simulink model "uuv_depth_control"  (R2021a)
settings: Solver=ode1  StartTime=0  StopTime=1000  FixedStep=0.1  RelTol=1e-3
undefined symbols (not defined in the file or in its folder): sigbuilder_block
(part 2 of 2)

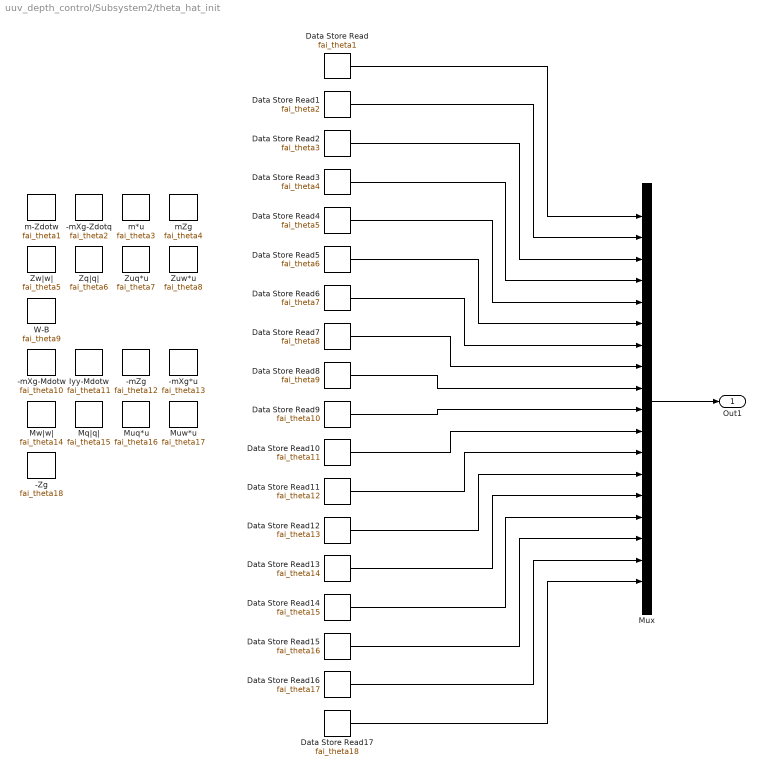
== system uuv_depth_control/Subsystem2/theta_hat_init ==
  -Zg : DataStoreMemory  DataStoreName=fai_theta18  ReadBeforeWriteMsg=warning  WriteAfterWriteMsg=warning  WriteAfterReadMsg=warning  InitialValue=-0.0196000000000000  ShowAdditionalParam=off
  -mXg*u : DataStoreMemory  DataStoreName=fai_theta13  ReadBeforeWriteMsg=warning  WriteAfterWriteMsg=warning  WriteAfterReadMsg=warning  ShowAdditionalParam=off
  -mXg-Mdotw : DataStoreMemory  DataStoreName=fai_theta10  ReadBeforeWriteMsg=warning  WriteAfterWriteMsg=warning  WriteAfterReadMsg=warning  InitialValue=1.93000000000000  ShowAdditionalParam=off
  -mXg-Zdotq : DataStoreMemory  DataStoreName=fai_theta2  ReadBeforeWriteMsg=warning  WriteAfterWriteMsg=warning  WriteAfterReadMsg=warning  InitialValue=1.930000000000000  ShowAdditionalParam=off
  -mZg : DataStoreMemory  DataStoreName=fai_theta12  ReadBeforeWriteMsg=warning  WriteAfterWriteMsg=warning  WriteAfterReadMsg=warning  InitialValue=-0.597408000000000  ShowAdditionalParam=off
  Data Store Read : DataStoreRead  DataStoreName=fai_theta1  IndexOptions=Index vector (dialog)  Indices=1  OutputSizes=1
  Data Store Read1 : DataStoreRead  DataStoreName=fai_theta2  IndexOptions=Index vector (dialog)  Indices=1  OutputSizes=1
  Data Store Read10 : DataStoreRead  DataStoreName=fai_theta11  IndexOptions=Index vector (dialog)  Indices=1  OutputSizes=1
  Data Store Read11 : DataStoreRead  DataStoreName=fai_theta12  IndexOptions=Index vector (dialog)  Indices=1  OutputSizes=1
  Data Store Read12 : DataStoreRead  DataStoreName=fai_theta13  IndexOptions=Index vector (dialog)  Indices=1  OutputSizes=1
  Data Store Read13 : DataStoreRead  DataStoreName=fai_theta14  IndexOptions=Index vector (dialog)  Indices=1  OutputSizes=1
  Data Store Read14 : DataStoreRead  DataStoreName=fai_theta15  IndexOptions=Index vector (dialog)  Indices=1  OutputSizes=1
  Data Store Read15 : DataStoreRead  DataStoreName=fai_theta16  IndexOptions=Index vector (dialog)  Indices=1  OutputSizes=1
  Data Store Read16 : DataStoreRead  DataStoreName=fai_theta17  IndexOptions=Index vector (dialog)  Indices=1  OutputSizes=1
  Data Store Read17 : DataStoreRead  DataStoreName=fai_theta18  IndexOptions=Index vector (dialog)  Indices=1  OutputSizes=1
  Data Store Read2 : DataStoreRead  DataStoreName=fai_theta3  IndexOptions=Index vector (dialog)  Indices=1  OutputSizes=1
  Data Store Read3 : DataStoreRead  DataStoreName=fai_theta4  IndexOptions=Index vector (dialog)  Indices=1  OutputSizes=1
  Data Store Read4 : DataStoreRead  DataStoreName=fai_theta5  IndexOptions=Index vector (dialog)  Indices=1  OutputSizes=1
  Data Store Read5 : DataStoreRead  DataStoreName=fai_theta6  IndexOptions=Index vector (dialog)  Indices=1  OutputSizes=1
  Data Store Read6 : DataStoreRead  DataStoreName=fai_theta7  IndexOptions=Index vector (dialog)  Indices=1  OutputSizes=1
  Data Store Read7 : DataStoreRead  DataStoreName=fai_theta8  IndexOptions=Index vector (dialog)  Indices=1  OutputSizes=1
  Data Store Read8 : DataStoreRead  DataStoreName=fai_theta9  IndexOptions=Index vector (dialog)  Indices=1  OutputSizes=1
  Data Store Read9 : DataStoreRead  DataStoreName=fai_theta10  IndexOptions=Index vector (dialog)  Indices=1  OutputSizes=1
  Iyy-Mdotw : DataStoreMemory  DataStoreName=fai_theta11  ReadBeforeWriteMsg=warning  WriteAfterWriteMsg=warning  WriteAfterReadMsg=warning  InitialValue=8.330000000000000  ShowAdditionalParam=off
  Mq|q| : DataStoreMemory  DataStoreName=fai_theta15  ReadBeforeWriteMsg=warning  WriteAfterWriteMsg=warning  WriteAfterReadMsg=warning  InitialValue=-9.40000000000000  ShowAdditionalParam=off
  Muq*u : DataStoreMemory  DataStoreName=fai_theta16  ReadBeforeWriteMsg=warning  WriteAfterWriteMsg=warning  WriteAfterReadMsg=warning  InitialValue=-1  ShowAdditionalParam=off
  Muw*u : DataStoreMemory  DataStoreName=fai_theta17  ReadBeforeWriteMsg=warning  WriteAfterWriteMsg=warning  WriteAfterReadMsg=warning  InitialValue=12  ShowAdditionalParam=off
  Mux : Mux  Inputs=18
  Mw|w| : DataStoreMemory  DataStoreName=fai_theta14  ReadBeforeWriteMsg=warning  WriteAfterWriteMsg=warning  WriteAfterReadMsg=warning  InitialValue=3.18000000000000  ShowAdditionalParam=off
  W-B : DataStoreMemory  DataStoreName=fai_theta9  ReadBeforeWriteMsg=warning  WriteAfterWriteMsg=warning  WriteAfterReadMsg=warning  InitialValue=-9  ShowAdditionalParam=off
  Zq|q| : DataStoreMemory  DataStoreName=fai_theta6  ReadBeforeWriteMsg=warning  WriteAfterWriteMsg=warning  WriteAfterReadMsg=warning  InitialValue=-0.632000000000000  ShowAdditionalParam=off
  Zuq*u : DataStoreMemory  DataStoreName=fai_theta7  ReadBeforeWriteMsg=warning  WriteAfterWriteMsg=warning  WriteAfterReadMsg=warning  InitialValue=-2.61000000000000  ShowAdditionalParam=off
  Zuw*u : DataStoreMemory  DataStoreName=fai_theta8  ReadBeforeWriteMsg=warning  WriteAfterWriteMsg=warning  WriteAfterReadMsg=warning  InitialValue=-14.3000000000000  ShowAdditionalParam=off
  Zw|w| : DataStoreMemory  DataStoreName=fai_theta5  ReadBeforeWriteMsg=warning  WriteAfterWriteMsg=warning  WriteAfterReadMsg=warning  InitialValue=-131  ShowAdditionalParam=off
  m*u : DataStoreMemory  DataStoreName=fai_theta3  ReadBeforeWriteMsg=warning  WriteAfterWriteMsg=warning  WriteAfterReadMsg=warning  InitialValue=15.2400000000000  ShowAdditionalParam=off
  m-Zdotw : DataStoreMemory  DataStoreName=fai_theta1  ReadBeforeWriteMsg=warning  WriteAfterWriteMsg=warning  WriteAfterReadMsg=warning  InitialValue=65.980000000000000  ShowAdditionalParam=off
  mZg : DataStoreMemory  DataStoreName=fai_theta4  ReadBeforeWriteMsg=warning  WriteAfterWriteMsg=warning  WriteAfterReadMsg=warning  InitialValue=0.597408000000000  ShowAdditionalParam=off
  Out1 : Outport
  wires:
  Mux/1 -> Out1/1
  Data Store Read/1 -> Mux/1
  Data Store Read3/1 -> Mux/4
  Data Store Read8/1 -> Mux/9
  Data Store Read5/1 -> Mux/6
  Data Store Read10/1 -> Mux/11
  Data Store Read4/1 -> Mux/5
  Data Store Read15/1 -> Mux/16
  Data Store Read12/1 -> Mux/13
  Data Store Read1/1 -> Mux/2
  Data Store Read14/1 -> Mux/15
  Data Store Read9/1 -> Mux/10
  Data Store Read7/1 -> Mux/8
  Data Store Read13/1 -> Mux/14
  Data Store Read2/1 -> Mux/3
  Data Store Read6/1 -> Mux/7
  Data Store Read17/1 -> Mux/18
  Data Store Read11/1 -> Mux/12
  Data Store Read16/1 -> Mux/17

== system uuv_depth_control/Subsystem4/cmd ==
  Add : Sum
  Cmd Depth : Subsystem  Tag=STV Subsys  LoadFcn=sigbuilder_block('load');  StartFcn=sigbuilder_block('start');  StopFcn=sigbuilder_block('stop');  ClipboardFcn=sigbuilder_block('clipboard');  mask(Sigbuilder block){tuvar=[0:10]}
      mask help: Simulink:masks:SigbuilderBlock_MD
      mask init:
      | if ~strcmp(get_param(bdroot(gcbh),'SimulationStatus'),'stopped') tuvar = sigbuilder_block('maskInit'); end
      settings: CopyFcn=sigbuilder_block('copy');  DeleteFcn=sigbuilder_block('delete');  ModelCloseFcn=sigbuilder_block('modelClose');  PreSaveFcn=sigbuilder_block('preSave');  PauseFcn=sigbuilder_block('pause');  ContinueFcn=sigbuilder_block('continue');  NameChangeFcn=sigbuilder_block('namechange');  OpenFcn=sigbuilder_block('open',[361.8 75 550.8 375 ]);  CloseFcn=sigbuilder_block('close');
      mask Display: plot(0, 0, 100, 100,[2, 2, 32, 32, 2], [68, 8, 8, 68, 68],[32, 2], [38, 38], [32, 19, 2],[53, 60, 44], [32, 17, 17, 2],[16, 16, 31, 31]);txt = getActiveGroup(gcbh);text(2, 100, txt,'verticalAlignment', 'top');
  Cmd theta : Subsystem  Tag=STV Subsys  LoadFcn=sigbuilder_block('load');  StartFcn=sigbuilder_block('start');  StopFcn=sigbuilder_block('stop');  ClipboardFcn=sigbuilder_block('clipboard');  mask(Sigbuilder block){tuvar=[0:10]}
      mask help: Simulink:masks:SigbuilderBlock_MD
      mask init:
      | if ~strcmp(get_param(bdroot(gcbh),'SimulationStatus'),'stopped') tuvar = sigbuilder_block('maskInit'); end
      settings: CopyFcn=sigbuilder_block('copy');  DeleteFcn=sigbuilder_block('delete');  ModelCloseFcn=sigbuilder_block('modelClose');  PreSaveFcn=sigbuilder_block('preSave');  PauseFcn=sigbuilder_block('pause');  ContinueFcn=sigbuilder_block('continue');  NameChangeFcn=sigbuilder_block('namechange');  OpenFcn=sigbuilder_block('open',[313.2 49.2 550.8 400.8 ]);  CloseFcn=sigbuilder_block('close');
      mask Display: plot(0, 0, 100, 100,[2, 2, 32, 32, 2], [68, 8, 8, 68, 68],[32, 2], [38, 38], [32, 19, 2],[53, 60, 44], [32, 17, 17, 2],[16, 16, 31, 31]);txt = getActiveGroup(gcbh);text(2, 100, txt,'verticalAlignment', 'top');
  Constant1 : Constant  Value=-1
  Constant2 : Constant  Value=0
  Constant3 : Constant
  Constant4 : Constant  Value=0
  Signal Generator : SignalGenerator  Amplitude=3  Frequency=0.1  Units=rad/sec
  Switch : Switch  Criteria=u2 > Threshold
  Switch1 : Switch  Criteria=u2 > Threshold
  Out1 : Outport
  Out2 : Outport  Port=2
  wires:
  Cmd Depth/1(Signal 2) -> Add/2
  Cmd theta/1(Signal 1) -> Switch1/1
  Signal Generator/1 -> Switch/1
  Add/1 -> Out1/1  "cmd_z"
  Constant4/1 -> Switch/3
  Switch/1 -> Add/1
  Constant1/1 -> Switch/2
  Constant2/1 -> Switch1/3
  Constant3/1 -> Switch1/2
  Switch1/1 -> Out2/1  "cmd_theta"

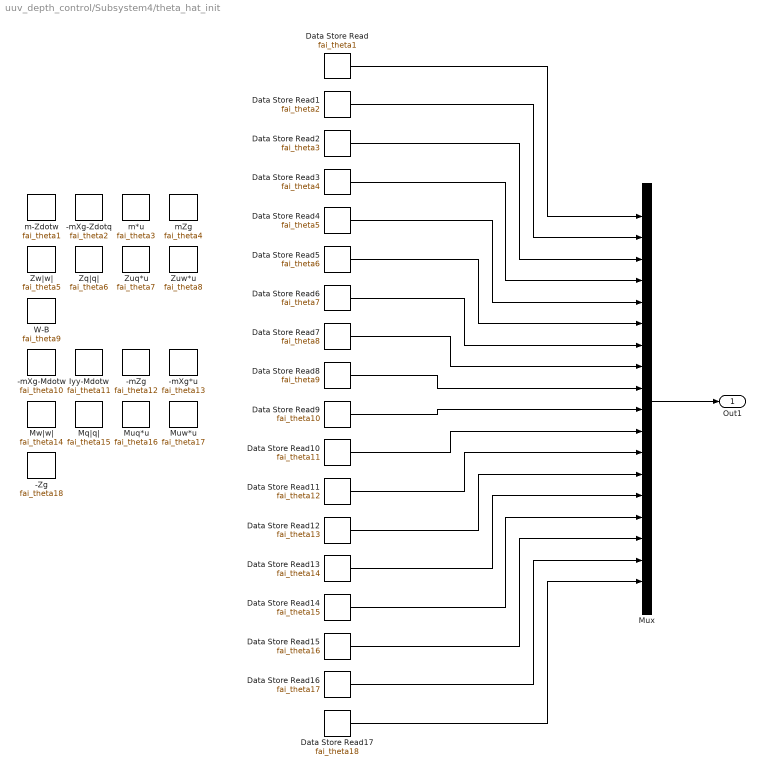
== system uuv_depth_control/Subsystem4/theta_hat_init ==
  -Zg : DataStoreMemory  DataStoreName=fai_theta18  ReadBeforeWriteMsg=warning  WriteAfterWriteMsg=warning  WriteAfterReadMsg=warning  InitialValue=-0.0196000000000000  ShowAdditionalParam=off
  -mXg*u : DataStoreMemory  DataStoreName=fai_theta13  ReadBeforeWriteMsg=warning  WriteAfterWriteMsg=warning  WriteAfterReadMsg=warning  ShowAdditionalParam=off
  -mXg-Mdotw : DataStoreMemory  DataStoreName=fai_theta10  ReadBeforeWriteMsg=warning  WriteAfterWriteMsg=warning  WriteAfterReadMsg=warning  InitialValue=1.93000000000000  ShowAdditionalParam=off
  -mXg-Zdotq : DataStoreMemory  DataStoreName=fai_theta2  ReadBeforeWriteMsg=warning  WriteAfterWriteMsg=warning  WriteAfterReadMsg=warning  InitialValue=1.930000000000000  ShowAdditionalParam=off
  -mZg : DataStoreMemory  DataStoreName=fai_theta12  ReadBeforeWriteMsg=warning  WriteAfterWriteMsg=warning  WriteAfterReadMsg=warning  InitialValue=-0.597408000000000  ShowAdditionalParam=off
  Data Store Read : DataStoreRead  DataStoreName=fai_theta1  IndexOptions=Index vector (dialog)  Indices=1  OutputSizes=1
  Data Store Read1 : DataStoreRead  DataStoreName=fai_theta2  IndexOptions=Index vector (dialog)  Indices=1  OutputSizes=1
  Data Store Read10 : DataStoreRead  DataStoreName=fai_theta11  IndexOptions=Index vector (dialog)  Indices=1  OutputSizes=1
  Data Store Read11 : DataStoreRead  DataStoreName=fai_theta12  IndexOptions=Index vector (dialog)  Indices=1  OutputSizes=1
  Data Store Read12 : DataStoreRead  DataStoreName=fai_theta13  IndexOptions=Index vector (dialog)  Indices=1  OutputSizes=1
  Data Store Read13 : DataStoreRead  DataStoreName=fai_theta14  IndexOptions=Index vector (dialog)  Indices=1  OutputSizes=1
  Data Store Read14 : DataStoreRead  DataStoreName=fai_theta15  IndexOptions=Index vector (dialog)  Indices=1  OutputSizes=1
  Data Store Read15 : DataStoreRead  DataStoreName=fai_theta16  IndexOptions=Index vector (dialog)  Indices=1  OutputSizes=1
  Data Store Read16 : DataStoreRead  DataStoreName=fai_theta17  IndexOptions=Index vector (dialog)  Indices=1  OutputSizes=1
  Data Store Read17 : DataStoreRead  DataStoreName=fai_theta18  IndexOptions=Index vector (dialog)  Indices=1  OutputSizes=1
  Data Store Read2 : DataStoreRead  DataStoreName=fai_theta3  IndexOptions=Index vector (dialog)  Indices=1  OutputSizes=1
  Data Store Read3 : DataStoreRead  DataStoreName=fai_theta4  IndexOptions=Index vector (dialog)  Indices=1  OutputSizes=1
  Data Store Read4 : DataStoreRead  DataStoreName=fai_theta5  IndexOptions=Index vector (dialog)  Indices=1  OutputSizes=1
  Data Store Read5 : DataStoreRead  DataStoreName=fai_theta6  IndexOptions=Index vector (dialog)  Indices=1  OutputSizes=1
  Data Store Read6 : DataStoreRead  DataStoreName=fai_theta7  IndexOptions=Index vector (dialog)  Indices=1  OutputSizes=1
  Data Store Read7 : DataStoreRead  DataStoreName=fai_theta8  IndexOptions=Index vector (dialog)  Indices=1  OutputSizes=1
  Data Store Read8 : DataStoreRead  DataStoreName=fai_theta9  IndexOptions=Index vector (dialog)  Indices=1  OutputSizes=1
  Data Store Read9 : DataStoreRead  DataStoreName=fai_theta10  IndexOptions=Index vector (dialog)  Indices=1  OutputSizes=1
  Iyy-Mdotw : DataStoreMemory  DataStoreName=fai_theta11  ReadBeforeWriteMsg=warning  WriteAfterWriteMsg=warning  WriteAfterReadMsg=warning  InitialValue=8.330000000000000  ShowAdditionalParam=off
  Mq|q| : DataStoreMemory  DataStoreName=fai_theta15  ReadBeforeWriteMsg=warning  WriteAfterWriteMsg=warning  WriteAfterReadMsg=warning  InitialValue=-9.40000000000000  ShowAdditionalParam=off
  Muq*u : DataStoreMemory  DataStoreName=fai_theta16  ReadBeforeWriteMsg=warning  WriteAfterWriteMsg=warning  WriteAfterReadMsg=warning  InitialValue=-1  ShowAdditionalParam=off
  Muw*u : DataStoreMemory  DataStoreName=fai_theta17  ReadBeforeWriteMsg=warning  WriteAfterWriteMsg=warning  WriteAfterReadMsg=warning  InitialValue=12  ShowAdditionalParam=off
  Mux : Mux  Inputs=18
  Mw|w| : DataStoreMemory  DataStoreName=fai_theta14  ReadBeforeWriteMsg=warning  WriteAfterWriteMsg=warning  WriteAfterReadMsg=warning  InitialValue=3.18000000000000  ShowAdditionalParam=off
  W-B : DataStoreMemory  DataStoreName=fai_theta9  ReadBeforeWriteMsg=warning  WriteAfterWriteMsg=warning  WriteAfterReadMsg=warning  InitialValue=-9  ShowAdditionalParam=off
  Zq|q| : DataStoreMemory  DataStoreName=fai_theta6  ReadBeforeWriteMsg=warning  WriteAfterWriteMsg=warning  WriteAfterReadMsg=warning  InitialValue=-0.632000000000000  ShowAdditionalParam=off
  Zuq*u : DataStoreMemory  DataStoreName=fai_theta7  ReadBeforeWriteMsg=warning  WriteAfterWriteMsg=warning  WriteAfterReadMsg=warning  InitialValue=-2.61000000000000  ShowAdditionalParam=off
  Zuw*u : DataStoreMemory  DataStoreName=fai_theta8  ReadBeforeWriteMsg=warning  WriteAfterWriteMsg=warning  WriteAfterReadMsg=warning  InitialValue=-14.3000000000000  ShowAdditionalParam=off
  Zw|w| : DataStoreMemory  DataStoreName=fai_theta5  ReadBeforeWriteMsg=warning  WriteAfterWriteMsg=warning  WriteAfterReadMsg=warning  InitialValue=-131  ShowAdditionalParam=off
  m*u : DataStoreMemory  DataStoreName=fai_theta3  ReadBeforeWriteMsg=warning  WriteAfterWriteMsg=warning  WriteAfterReadMsg=warning  InitialValue=15.2400000000000  ShowAdditionalParam=off
  m-Zdotw : DataStoreMemory  DataStoreName=fai_theta1  ReadBeforeWriteMsg=warning  WriteAfterWriteMsg=warning  WriteAfterReadMsg=warning  InitialValue=65.980000000000000  ShowAdditionalParam=off
  mZg : DataStoreMemory  DataStoreName=fai_theta4  ReadBeforeWriteMsg=warning  WriteAfterWriteMsg=warning  WriteAfterReadMsg=warning  InitialValue=0.597408000000000  ShowAdditionalParam=off
  Out1 : Outport
  wires:
  Mux/1 -> Out1/1
  Data Store Read/1 -> Mux/1
  Data Store Read3/1 -> Mux/4
  Data Store Read8/1 -> Mux/9
  Data Store Read5/1 -> Mux/6
  Data Store Read10/1 -> Mux/11
  Data Store Read4/1 -> Mux/5
  Data Store Read15/1 -> Mux/16
  Data Store Read12/1 -> Mux/13
  Data Store Read1/1 -> Mux/2
  Data Store Read14/1 -> Mux/15
  Data Store Read9/1 -> Mux/10
  Data Store Read7/1 -> Mux/8
  Data Store Read13/1 -> Mux/14
  Data Store Read2/1 -> Mux/3
  Data Store Read6/1 -> Mux/7
  Data Store Read17/1 -> Mux/18
  Data Store Read11/1 -> Mux/12
  Data Store Read16/1 -> Mux/17

== system uuv_depth_control/speed_cintrol/Kinetic model ==
  ur|ur| : Inport
  tao_u : Inport  Port=2
  Input : Inport  Port=3
  Add2 : Sum  Inputs=+++
  Constant5 : Constant  Value=-1
  Constant6 : Constant
  Divide : Product  Inputs=*/
  MATLAB Function : MATLAB Function  TreatAsAtomicUnit=on
  Matrix Multiply4 : Product  Multiplication=Matrix(*)
  Switch1 : Switch  Criteria=u2 > Threshold
  dot_ur : Outport
  wires:
  MATLAB Function/1(gama_true) -> Divide/2  "gama_true"
  MATLAB Function/2(beta_true) -> Matrix Multiply4/1  "beta_true"
  MATLAB Function/3(delta_true) -> Add2/3  "delta_true"
  Matrix Multiply4/1 -> Add2/2
  tao_u/1 -> Divide/1
  Divide/1 -> Add2/1
  Add2/1 -> dot_ur/1  "dot_ur"
  ur|ur|/1 -> Matrix Multiply4/2
  Input/1 -> Switch1/2
  Constant6/1 -> Switch1/1
  Constant5/1 -> Switch1/3
  Switch1/1 -> MATLAB Function/1(delta_u)  "delta_u"

== system uuv_depth_control/speed_cintrol/controller ==
  ur|ur| : Inport
  dot_ud : Inport  Port=2
  Z1 : Inport  Port=3
  Add : Sum  Inputs=----+
  Add4 : Sum  Inputs=+---+
  Constant1 : Constant  Value=-1
  Constant5 : Constant
  Gain : Gain  Gain=0.07
  Integrator4 : Integrator
  Integrator6 : Integrator  InitialCondition=-0.054
  Integrator7 : Integrator  InitialCondition=34.9
  Matrix Multiply{4,6..8} (4 alike) : Product  Multiplication=Matrix(*)
  Switch1 : Switch  Criteria=u2 > Threshold
  eta1 : Gain  Gain=0.01
  k1 : Gain  Gain=3
  tao_u : Outport
  wires:
  ur|ur|/1 -> Matrix Multiply4/1, Matrix Multiply7/1  "ur|ur|"
  Constant1/1 -> Switch1/3
  Switch1/1 -> eta1/1
  Integrator7/1 -> Matrix Multiply8/2  "gama_hat"
  Constant5/1 -> Switch1/1
  Matrix Multiply7/1 -> Add/4, Add4/2  "beta_hat*ur|ur|"
  Integrator6/1 -> Matrix Multiply7/2  "beta_hat"
  Integrator4/1 -> Add/3, Add4/3  "dot_uf_hat"
  Add4/1 -> Matrix Multiply8/1
  k1/1 -> Add/2, Add4/4  "k1Z1"
  eta1/1 -> Add4/5, Add/1  "滑膜项"
  Gain/1 -> Matrix Multiply4/2, Matrix Multiply6/1, Integrator4/1  "dd_uf_hat"
  Matrix Multiply6/1 -> Integrator7/1  "dot_gama_hat"
  Matrix Multiply4/1 -> Integrator6/1  "dot_beta_hat"
  Add/1 -> Matrix Multiply6/2  "Fai"
  dot_ud/1 -> Add/5, Add4/1
  Matrix Multiply8/1 -> tao_u/1  "tao_u"
  Z1/1 -> Switch1/2, k1/1, Gain/1

== system uuv_depth_control/Subsystem/cmd/Cmd Depth ==
  Demux : Demux  Tag=STV Demux  Outputs=1
      settings: DisplayOption=none
  FromWs : FromWorkspace  Tag=STV FromWs  VariableName=tuvar
      SigBuilderData=|
      | common.afterFinalStr = 'Extrapolate'
      | common.sampleTime = 0
      | dataSet.timeRange = [0 3000]
      | dataSet.name = 'Group 1'
      | sbobj.Groups.Name = 'Group 1'
      | sbobj.Groups.Signals.Name = 'Signal 1'
      | sbobj.Groups.Signals.XData = [0 500 1500 2000 3000]
      | sbobj.Groups.Signals.YData = [30 30 30 30 30]
      | sbobj.Groups.TimeRange = [0 3000]
  Signal 1 : Outport  Tag=STV Outport
  wires:
  Demux/1 -> Signal 1/1
  FromWs/1 -> Demux/1

== system uuv_depth_control/Subsystem/cmd/Cmd theta ==
  Demux : Demux  Tag=STV Demux  Outputs=1
      settings: DisplayOption=none
  FromWs : FromWorkspace  Tag=STV FromWs  VariableName=tuvar
      SigBuilderData=|
      | common.afterFinalStr = 'Extrapolate'
      | common.sampleTime = 0
      | dataSet.timeRange = [0 200]
      | dataSet.name = 'Group 1'
      | sbobj.Groups.Name = 'Group 1'
      | sbobj.Groups.Signals.Name = 'Signal 1'
      | sbobj.Groups.Signals.XData = [0 30 80 200]
      | sbobj.Groups.Signals.YData = [0 7 7 7]
      | sbobj.Groups.TimeRange = [0 200]
  Signal 1 : Outport  Tag=STV Outport
  wires:
  Demux/1 -> Signal 1/1
  FromWs/1 -> Demux/1

== system uuv_depth_control/Subsystem1/cmd/Cmd Depth ==
  Demux : Demux  Tag=STV Demux  Outputs=1
      settings: DisplayOption=none
  FromWs : FromWorkspace  Tag=STV FromWs  VariableName=tuvar
      SigBuilderData=|
      | common.afterFinalStr = 'Extrapolate'
      | common.sampleTime = 0
      | dataSet.timeRange = [0 1000]
      | dataSet.name = 'Group 1'
      | sbobj.Groups.Name = 'Group 1'
      | sbobj.Groups.Signals.Name = 'Signal 1'
      | sbobj.Groups.Signals.XData = [0 1000]
      | sbobj.Groups.Signals.YData = [40 40]
      | sbobj.Groups.TimeRange = [0 1000]
  Signal 1 : Outport  Tag=STV Outport
  wires:
  FromWs/1 -> Demux/1
  Demux/1 -> Signal 1/1

== system uuv_depth_control/Subsystem1/cmd/Cmd theta ==
  Demux : Demux  Tag=STV Demux  Outputs=1
      settings: DisplayOption=none
  FromWs : FromWorkspace  Tag=STV FromWs  VariableName=tuvar
      SigBuilderData=|
      | common.afterFinalStr = 'Extrapolate'
      | common.sampleTime = 0
      | dataSet.timeRange = [0 1000]
      | dataSet.name = 'Group 1'
      | sbobj.Groups.Name = 'Group 1'
      | sbobj.Groups.Signals.Name = 'Signal 1'
      | sbobj.Groups.Signals.XData = [0 300 500 1000]
      | sbobj.Groups.Signals.YData = [3 3 3 3]
      | sbobj.Groups.TimeRange = [0 1000]
  Signal 1 : Outport  Tag=STV Outport
  wires:
  FromWs/1 -> Demux/1
  Demux/1 -> Signal 1/1

== system uuv_depth_control/Subsystem2/cmd/Cmd Depth ==
  Demux : Demux  Tag=STV Demux  Outputs=1
      settings: DisplayOption=none
  FromWs : FromWorkspace  Tag=STV FromWs  VariableName=tuvar
      SigBuilderData=|
      | common.afterFinalStr = 'Extrapolate'
      | common.sampleTime = 0
      | dataSet.timeRange = [0 1000]
      | dataSet.name = 'Group 1'
      | sbobj.Groups.Name = 'Group 1'
      | sbobj.Groups.Signals.Name = 'Signal 2'
      | sbobj.Groups.Signals.XData = [0 50 500 1000]
      | sbobj.Groups.Signals.YData = [40 40 40 40]
      | sbobj.Groups.TimeRange = [0 1000]
  Signal 2 : Outport  Tag=STV Outport
  wires:
  FromWs/1 -> Demux/1
  Demux/1 -> Signal 2/1

== system uuv_depth_control/Subsystem2/cmd/Cmd theta ==
  Demux : Demux  Tag=STV Demux  Outputs=1
      settings: DisplayOption=none
  FromWs : FromWorkspace  Tag=STV FromWs  VariableName=tuvar
      SigBuilderData=|
      | common.afterFinalStr = 'Extrapolate'
      | common.sampleTime = 0
      | dataSet.timeRange = [0 1000]
      | dataSet.name = 'Group 1'
      | sbobj.Groups.Name = 'Group 1'
      | sbobj.Groups.Signals.Name = 'Signal 1'
      | sbobj.Groups.Signals.XData = [0 20 500 1000]
      | sbobj.Groups.Signals.YData = [3 3 3 3]
      | sbobj.Groups.TimeRange = [0 1000]
  Signal 1 : Outport  Tag=STV Outport
  wires:
  FromWs/1 -> Demux/1
  Demux/1 -> Signal 1/1

== system uuv_depth_control/Subsystem4/cmd/Cmd Depth ==
  Demux : Demux  Tag=STV Demux  Outputs=1
      settings: DisplayOption=none
  FromWs : FromWorkspace  Tag=STV FromWs  VariableName=tuvar
      SigBuilderData=|
      | common.afterFinalStr = 'Extrapolate'
      | common.sampleTime = 0
      | dataSet.timeRange = [0 1000]
      | dataSet.name = 'Group 1'
      | sbobj.Groups.Name = 'Group 1'
      | sbobj.Groups.Signals.Name = 'Signal 2'
      | sbobj.Groups.Signals.XData = [0 50 500 1000]
      | sbobj.Groups.Signals.YData = [0 40 40 40]
      | sbobj.Groups.TimeRange = [0 1000]
  Signal 2 : Outport  Tag=STV Outport
  wires:
  FromWs/1 -> Demux/1
  Demux/1 -> Signal 2/1

== system uuv_depth_control/Subsystem4/cmd/Cmd theta ==
  Demux : Demux  Tag=STV Demux  Outputs=1
      settings: DisplayOption=none
  FromWs : FromWorkspace  Tag=STV FromWs  VariableName=tuvar
      SigBuilderData=|
      | common.afterFinalStr = 'Extrapolate'
      | common.sampleTime = 0
      | dataSet.timeRange = [0 1000]
      | dataSet.name = 'Group 1'
      | sbobj.Groups.Name = 'Group 1'
      | sbobj.Groups.Signals.Name = 'Signal 1'
      | sbobj.Groups.Signals.XData = [0 20 500 1000]
      | sbobj.Groups.Signals.YData = [0 3 3 3]
      | sbobj.Groups.TimeRange = [0 1000]
  Signal 1 : Outport  Tag=STV Outport
  wires:
  FromWs/1 -> Demux/1
  Demux/1 -> Signal 1/1

== matlab function uuv_depth_control/Param1 ==
  data: J_theta_line1 output; J_theta_line2 output; u_sind output; M_uuv_inv_line1 output; M_uuv_inv_line2 output; tao_out output; fc_wq output; fd_wq output; fg_theta output; T_vector output; w input; q input; theta input; theta_hat input; tao_in input
function [J_theta_line1,J_theta_line2,u_sind,M_uuv_inv_line1,M_uuv_inv_line2,tao_out,fc_wq,fd_wq,fg_theta,T_vector]= Param(w,q,theta,theta_hat, tao_in)
auv.L1 = 0.35;
auv.L2 = 0.35;
auv.u = 0.5;
M_uuv_inv = inv([theta_hat(1),theta_hat(2);
                 theta_hat(10),theta_hat(11)]);
fc_wq = [theta_hat(3)*q+theta_hat(4)*q*q;
         theta_hat(12)*w*q+theta_hat(13)*q]; 
fd_wq = [theta_hat(5)*w*abs(w)+theta_hat(6)*q*abs(q)+theta_hat(7)*q+theta_hat(8)*w;
         theta_hat(14)*w*abs(w)+theta_hat(15)*q*abs(q)+theta_hat(16)*q+theta_hat(17)*w];
fg_theta = [cosd(theta)*theta_hat(9);
            sind(theta)*theta_hat(18)];
u_sind = [auv.u*sind(theta);0];

J_theta = [ cosd(theta),0 ; 0,1];
J_theta_line1= J_theta(1,:) ;
J_theta_line2= J_theta(2,:) ;

M_uuv_inv_line1 = M_uuv_inv(:,1);
M_uuv_inv_line2 = M_uuv_inv(:,2); 

tao_out = tao_in;
T_vector= inv([1,1;-auv.L1,auv.L2])*tao_in;
end

== matlab function uuv_depth_control/Fai1/MATLAB Function ==
  data: w_w_ input; Fai output size=[2 18]; w input; dotw input; q_q_ input; q input; dotq input; q_2 input; wq input; theta input; Fai_t output size=[18 2]
function [Fai,Fai_t] = fcn(w_w_, w, dotw, q_q_, q, dotq, q_2, wq, theta)
Fai_1 = [dotw,dotq,q,q_2,w_w_,q_q_,q,w,cosd(theta),0,0,0,0,0,0,0,0,0];
Fai_2 = [0,0,0,0,0,0,0,0,0,dotw,dotq,wq,q,w_w_,q_q_,q,w,sind(theta)];
Fai = [Fai_1;Fai_2];
Fai_t = [Fai_1;Fai_2]';
end

== matlab function uuv_depth_control/Kinetic model2/J_theta_connect ==
  data: in_1 input; out output size=[2 2]; in_2 input
function out = Link(in_1,in_2)

out = [in_1;in_2];

end

== matlab function uuv_depth_control/Kinetic model2/M_uuv_inv_link ==
  data: in_1 input; inv_out output size=[2 2]; in_2 input
function inv_out = Link(in_1,in_2)

inv_out = [in_1,in_2];

end

== matlab function uuv_depth_control/Param2 ==
  data: J_theta_line1 output; J_theta_line2 output; u_sind output; M_uuv_inv_line1 output; M_uuv_inv_line2 output; tao_out output; fc_wq output; fd_wq output; fg_theta output; T_vector output; w input; q input; theta input; tao_in input; u input
function [J_theta_line1,J_theta_line2,u_sind,M_uuv_inv_line1,M_uuv_inv_line2,tao_out,fc_wq,fd_wq,fg_theta,T_vector]= Param(w,q,theta,tao_in,u)

auv = Auv_param_true();

J_theta = [ cosd(theta),0 ; 0,1];
J_theta_line1= J_theta(1,:) ;
J_theta_line2= J_theta(2,:) ;

M_uuv_inv = inv([auv.m-auv.Zdotw,-auv.m*auv.xg-auv.Zdotq;-auv.m*auv.xg-auv.Mdotw,auv.Iyy-auv.Mdotq]);
M_uuv_inv_line1 = M_uuv_inv(:,1);
M_uuv_inv_line2 = M_uuv_inv(:,2); 
T_vector= inv([1,1;-auv.L1,auv.L2])*tao_in;
fc_wq = [auv.m*(u*q+auv.zg*q^2) ;
        -auv.m*(auv.zg*w*q+auv.xg*u*q)]; 
fd_wq = [(auv.Zww*w*abs(w)+auv.Zqq*q*abs(q)+auv.Zuq*u*q+u*w*u*w) ;
        (auv.Mww*w*abs(w)+auv.Mqq*q*abs(q)+auv.Muq*u*q+auv.Muw*u*w)];
fg_theta = [(auv.W-auv.B)*cosd(theta);
            -(auv.zg*auv.W-auv.zb*auv.B)*sind(theta)-(auv.xg*auv.W-auv.xb*auv.B)*cosd(theta)];
u_sind = [u*sind(theta);0];
tao_out = tao_in;

end

== matlab function uuv_depth_control/speed_cintrol/Kinetic model/MATLAB Function ==
  data: gama_true output; beta_true output; delta_true output; delta_u input
function [gama_true,beta_true,delta_true]= param(delta_u)
t = 0.1;    %推力减额系数
T_tao = 1;  %推力系数
auv = Auv_param_true;
gama_true = (auv.m-auv.Xdotu)/((1-t)*T_tao);%>0
beta_true = auv.Xuu/(auv.m-auv.Xdotu);             %<0
delta_true = delta_u/(auv.m-auv.Xdotu);

end

== matlab function uuv_depth_control/动力学模型1/MATLAB Function ==
  data: gama_true output; beta_true output; delta_true output; delta_u input
function [gama_true,beta_true,delta_true]= param(delta_u)
t = 0.1;    %推力减额系数
T_tao = 1;  %推力系数
auv = Auv_param_true;
gama_true = (auv.m-auv.Xdotu)/((1-t)*T_tao);%>0
beta_true = auv.Xuu/(auv.m-auv.Xdotu);             %<0
delta_true = delta_u/(auv.m-auv.Xdotu);

end

== matlab function uuv_depth_control/Subsystem2/MATLAB Function ==
  data: tao_in input; tao_out output
function tao_out = fcn(tao_in)
if tao_in(1) > 120
    tao_in(1) = 120;
end
if tao_in(1) < -120
    tao_in(1) = -120;
end
if tao_in(2) > 120
    tao_in(2) = 120;
end
if tao_in(2) < -120
    tao_in(2) = -120;
end
tao_out = tao_in;

== matlab function uuv_depth_control/Fai4/MATLAB Function ==
  data: w_w_ input; Fai output size=[2 18]; w input; dotw input; q_q_ input; q input; dotq input; q_2 input; wq input; theta input; Fai_t output size=[18 2]
function [Fai,Fai_t] = fcn(w_w_, w, dotw, q_q_, q, dotq, q_2, wq, theta)
Fai_1 = [dotw,dotq,q,q_2,w_w_,q_q_,q,w,cosd(theta),0,0,0,0,0,0,0,0,0];
Fai_2 = [0,0,0,0,0,0,0,0,0,dotw,dotq,wq,q,w_w_,q_q_,q,w,sind(theta)];
Fai = [Fai_1;Fai_2];
Fai_t = [Fai_1;Fai_2]';
end

== matlab function uuv_depth_control/Kinetic model4/J_theta_connect ==
  data: in_1 input; out output size=[2 2]; in_2 input
function out = Link(in_1,in_2)

out = [in_1;in_2];

end

== matlab function uuv_depth_control/Kinetic model4/M_uuv_inv_link ==
  data: in_1 input; inv_out output size=[2 2]; in_2 input
function inv_out = Link(in_1,in_2)

inv_out = [in_1,in_2];

end

== matlab function uuv_depth_control/Param4 ==
  data: J_theta_line1 output; J_theta_line2 output; u_sind output; M_uuv_inv_line1 output; M_uuv_inv_line2 output; tao_out output; fc_wq output; fd_wq output; fg_theta output; T_vector output; w input; q input; theta input; tao_in input
function [J_theta_line1,J_theta_line2,u_sind,M_uuv_inv_line1,M_uuv_inv_line2,tao_out,fc_wq,fd_wq,fg_theta,T_vector]= Param(w,q,theta,tao_in)

auv = Auv_param_true();

J_theta = [ cosd(theta),0 ; 0,1];
J_theta_line1= J_theta(1,:) ;
J_theta_line2= J_theta(2,:) ;

M_uuv_inv = inv([auv.m-auv.Zdotw,-auv.m*auv.xg-auv.Zdotq;-auv.m*auv.xg-auv.Mdotw,auv.Iyy-auv.Mdotq]);
M_uuv_inv_line1 = M_uuv_inv(:,1);
M_uuv_inv_line2 = M_uuv_inv(:,2); 
T_vector= inv([1,1;-auv.L1,auv.L2])*tao_in;
fc_wq = [auv.m*(auv.u*q+auv.zg*q^2) ;
        -auv.m*(auv.zg*w*q+auv.xg*auv.u*q)]; 
fd_wq = [(auv.Zww*w*abs(w)+auv.Zqq*q*abs(q)+auv.Zuq*auv.u*q+auv.u*w*auv.u*w) ;
        (auv.Mww*w*abs(w)+auv.Mqq*q*abs(q)+auv.Muq*auv.u*q+auv.Muw*auv.u*w)];
fg_theta = [(auv.W-auv.B)*cosd(theta);
            -(auv.zg*auv.W-auv.zb*auv.B)*sind(theta)-(auv.xg*auv.W-auv.xb*auv.B)*cosd(theta)];
u_sind = [auv.u*sind(theta);0];
tao_out = tao_in;

end

== matlab function uuv_depth_control/Kinetic model/J_theta_connect ==
  data: in_1 input; out output size=[2 2]; in_2 input
function out = Link(in_1,in_2)

out = [in_1;in_2];

end

== matlab function uuv_depth_control/Param ==
  data: J_theta_line1 output; J_theta_line2 output; u_sind output; M_uuv_inv_line1 output; M_uuv_inv_line2 output; tao_out output; fc_wq output; fd_wq output; fg_theta output; T_vector output; w input; q input; theta input; tao_in input
function [J_theta_line1,J_theta_line2,u_sind,M_uuv_inv_line1,M_uuv_inv_line2,tao_out,fc_wq,fd_wq,fg_theta,T_vector]= Param(w,q,theta,tao_in)

auv = Auv_param();

J_theta = [ cosd(theta),0 ; 0,1];
J_theta_line1= J_theta(1,:) ;
J_theta_line2= J_theta(2,:) ;

M_uuv_inv = inv([auv.m-auv.Zdotw,-auv.m*auv.xg-auv.Zdotq;-auv.m*auv.xg-auv.Mdotw,auv.Iyy-auv.Mdotq]);
M_uuv_inv_line1 = M_uuv_inv(:,1);
M_uuv_inv_line2 = M_uuv_inv(:,2); 
T_vector= inv([1,1;-auv.L1,auv.L2])*tao_in;
fc_wq = [auv.m*(auv.u*q+auv.zg*q^2) ;
        -auv.m*(auv.zg*w*q+auv.xg*auv.u*q)]; 
fd_wq = [(auv.Zww*w*abs(w)+auv.Zqq*q*abs(q)+auv.Zuq*auv.u*q+auv.u*w*auv.u*w) ;
        (auv.Mww*w*abs(w)+auv.Mqq*q*abs(q)+auv.Muq*auv.u*q+auv.Muw*auv.u*w)];
fg_theta = [(auv.W-auv.B)*cosd(theta);
            -(auv.zg*auv.W-auv.zb*auv.B)*sind(theta)-(auv.xg*auv.W-auv.xb*auv.B)*cosd(theta)];
u_sind = [auv.u*sind(theta);0];
tao_out = tao_in;

end

== matlab function uuv_depth_control/Kinetic model/M_uuv_inv_link ==
  data: in_1 input; inv_out output size=[2 2]; in_2 input; M_uuv output size=[2 2]
function [inv_out,M_uuv] = Link(in_1,in_2)

inv_out = [in_1,in_2];
M_uuv = inv(inv_out);

end

== matlab function uuv_depth_control/Fai2/MATLAB Function ==
  data: w_w_ input; Fai output size=[2 18]; w input; dotw input; q_q_ input; q input; dotq input; q_2 input; wq input; theta input; Fai_t output size=[18 2]
function [Fai,Fai_t] = fcn(w_w_, w, dotw, q_q_, q, dotq, q_2, wq, theta)
Fai_1 = [dotw,dotq,q,q_2,w_w_,q_q_,q,w,cosd(theta),0,0,0,0,0,0,0,0,0];
Fai_2 = [0,0,0,0,0,0,0,0,0,dotw,dotq,wq,q,w_w_,q_q_,q,w,sind(theta)];
Fai = [Fai_1;Fai_2];
Fai_t = [Fai_1;Fai_2]';
end

== matlab function uuv_depth_control/Kinetic model1/J_theta_connect ==
  data: in_1 input; out output size=[2 2]; in_2 input
function out = Link(in_1,in_2)

out = [in_1;in_2];

end

== matlab function uuv_depth_control/Kinetic model1/M_uuv_inv_link ==
  data: in_1 input; inv_out output size=[2 2]; in_2 input
function inv_out = Link(in_1,in_2)

inv_out = [in_1,in_2];

end
